simulink model "AUAV3_WITH_SLUGS_SENSOR_AND_CONTROLLER"  (Simulink 8.5)
settings: Solver=FixedStepDiscrete  StartTime=0.0  StopTime=10.0  FixedStep=T  RelTol=1e-3
PreLoadFcn:
  | T = 0.0025;
  | MavlinkBus;
  | 
  | % Baro Altitude Computation
  | % =========================
  | basePressure = 98192.64;
  | baseTemp = 288.215;
  | lapseRate = -0.00198122;
  | baseHeight = 0;
  | 
  | mcuInit
values from neighbouring files (symbols this model uses):
  apSampleTime = 0.01    [mcuInit.m]
  latlong_WP = 1    [mcuInit.m]
  mavlink_gps_raw_int_t = Simulink.Bus    [MavlinkBus.m]    (also in MavlinkBusMarcello.m)
  mavlink_raw_imu_t = Simulink.Bus    [MavlinkBus.m]    (also in MavlinkBusMarcello.m)
  mavlink_scaled_pressure_t = Simulink.Bus    [MavlinkBus.m]    (also in MavlinkBusMarcello.m)
  mavlink_sys_status_t = Simulink.Bus    [MavlinkBus.m]    (also in MavlinkBusMarcello.m)
  Xpoints = [0 0]    [mcuInit.m]
  Ypoints = [0 0]    [mcuInit.m]
  Zpoints = [0 0]    [mcuInit.m]
undefined symbols (not defined in the file or in its folder): A0, A14, A15, A2, A3, A5, A6, accBiasRateLimit, altLatLon, B0, bankCommandLimit, barAdjust, baroCutoff, baroCutTemp, C3, cubeAccelGain16405, cubeGyroGain16405, cubeMagGain16405, D0, D11, D13, D8, daLimit, data, daTrimMax, daTrimMin, deLimit, deTrimMax, deTrimMin, drLimit, drTrimMax, drTrimMin, dtLimit, dtTrimMax, dtTrimMin, F2, F3, G0, G15, gaind, GS_location, gyroBiasRateLimit, IC1max, IPStar, ISA_g, maxAcc, MaxDwnPthStar, maxDynPressure, maxEta, OC1max, P112, P127, P16, P21, P30, P31, P51, P64, P72, P75 ... (+39)
undefined symbols (not defined in the file): baroOffset, baroScale, barTGain1, barTGain2, barTMean1, barTMean2, bda, bde, bdr, bdt, bICda, bICde, bICdr, bICdt, derivativesConstant, lowRateSensorCutoff, mainSensorCutoff, mda, mde, mdr, mdt, mICda, mICde, mICdr, mICdt, pitotOffset, pitotScale, pitTGain1, pitTGain2, pitTMean1, pitTMean2, powerOffset, powerScale, pressureSensorCutoff, tempOffset, tempScale, vzCutoff, xCutoff, yCutoff
libraries: MCHP_Blockset x147, simulink x78, SLUGS_Library x31, aerolibconvert2 x6, aerolibutil x4, aerolibtransform2 x3, dspmtrx3 x2, aerolibobsolete x2
(part 12 of 12)

== matlab function Sensor Data [updated 4.28.16]/Sensor Suite/ADIS16405 Signal Cond /3D Tustin Lowpass, Auto Initial Condition/Embedded MATLAB Function1 ==
  data: u input double; y output double; T input double; f input double
function y = fcn(u,T,f)
% This block supports an embeddable subset of the MATLAB language.
% See the help menu for details. 

persistent a
persistent b
persistent y_km1
persistent u_km1
if isempty(a)
    %tf = [T*omega/(2+T*omega) T*omega/(2+T*omega)],[1 (T*omega-2)/(T*omega+2)]
    %tf = [a a],[1 -b]
    omega = 2*pi*f;
    a=T*omega/(2+T*omega);
    b=-(T*omega-2)/(T*omega+2);
    y_km1=u;
    u_km1=u;
end

y = a*(u+u_km1)+b*y_km1;
y_km1=y;
u_km1=u;

== matlab function Trim Vals [updated 4.28.16]/Control Surface Input/2 sec  tau/Embedded MATLAB Function ==
  data: u input double; y output double; T input double; f input double
function y = fcn(u,T,f)
% This block supports an embeddable subset of the MATLAB language.
% See the help menu for details. 

persistent a
persistent b
persistent y_km1
persistent u_km1
if isempty(a)
    %tf = [T*omega/(2+T*omega) T*omega/(2+T*omega)],[1 (T*omega-2)/(T*omega+2)]
    %tf = [a a],[1 -b]
    omega = 2*pi*f;
    a=T*omega/(2+T*omega);
    b=-(T*omega-2)/(T*omega+2);
    y_km1=u;
    u_km1=u;
end

y = a*(u+u_km1)+b*y_km1;
y_km1=y;
u_km1=u;

== matlab function Trim Vals [updated 4.28.16]/Control Surface Input/2 sec  tau1/Embedded MATLAB Function ==
  data: u input double; y output double; T input double; f input double
function y = fcn(u,T,f)
% This block supports an embeddable subset of the MATLAB language.
% See the help menu for details. 

persistent a
persistent b
persistent y_km1
persistent u_km1
if isempty(a)
    %tf = [T*omega/(2+T*omega) T*omega/(2+T*omega)],[1 (T*omega-2)/(T*omega+2)]
    %tf = [a a],[1 -b]
    omega = 2*pi*f;
    a=T*omega/(2+T*omega);
    b=-(T*omega-2)/(T*omega+2);
    y_km1=u;
    u_km1=u;
end

y = a*(u+u_km1)+b*y_km1;
y_km1=y;
u_km1=u;

== matlab function Sensor Data [updated 4.28.16]/Sensor Suite/ADIS16405 Signal Cond /3D Tustin Lowpass, Auto Initial Condition/Embedded MATLAB Function2 ==
  data: u input double; y output double; T input double; f input double
function y = fcn(u,T,f)
% This block supports an embeddable subset of the MATLAB language.
% See the help menu for details. 

persistent a
persistent b
persistent y_km1
persistent u_km1
if isempty(a)
    %tf = [T*omega/(2+T*omega) T*omega/(2+T*omega)],[1 (T*omega-2)/(T*omega+2)]
    %tf = [a a],[1 -b]
    omega = 2*pi*f;
    a=T*omega/(2+T*omega);
    b=-(T*omega-2)/(T*omega+2);
    y_km1=u;
    u_km1=u;
end

y = a*(u+u_km1)+b*y_km1;
y_km1=y;
u_km1=u;

== matlab function Trim Vals [updated 4.28.16]/Mean Filter the Transition/Buffer Failsafe Channel ==
  data: latest input double; history output double
function history = bufferICValues(latest)
% This block supports an embeddable subset of the MATLAB language.
% See the help menu for details. 

persistent oldValues;

if isempty(oldValues)
    oldValues = uint16([0 0 0 0 0 0 0]);
end

history = uint16([0 0 0 0 0 0 0]);

for i=7:-1:2
    oldValues(i) = oldValues(i-1);
	history(i) = oldValues(i-1);
end
	
oldValues(1) = latest;
history(1) = latest;

== matlab function Sensor Data [updated 4.28.16]/Sensor Suite/ADIS16405 Signal Cond /3D Tustin Lowpass, Auto Initial Condition/myMux Fun ==
  data: u1 input double; y output double; u2 input double; u3 input double
function y = myMux3(u1, u2, u3)
% This block supports an embeddable subset of the MATLAB language.
% See the help menu for details. 

y = [u1(1); u2(1); u3(1)];

== matlab function Sensor Data [updated 4.28.16]/Sensor Suite/ADIS16405 Signal Cond /3D Tustin Lowpass, Auto Initial Condition1/Embedded MATLAB Function ==
  data: u input double; y output double; T input double; f input double
function y = fcn(u,T,f)
% This block supports an embeddable subset of the MATLAB language.
% See the help menu for details. 

persistent a
persistent b
persistent y_km1
persistent u_km1
if isempty(a)
    %tf = [T*omega/(2+T*omega) T*omega/(2+T*omega)],[1 (T*omega-2)/(T*omega+2)]
    %tf = [a a],[1 -b]
    omega = 2*pi*f;
    a=T*omega/(2+T*omega);
    b=-(T*omega-2)/(T*omega+2);
    y_km1=u;
    u_km1=u;
end

y = a*(u+u_km1)+b*y_km1;
y_km1=y;
u_km1=u;

== matlab function Sensor Data [updated 4.28.16]/Sensor Suite/ADIS16405 Signal Cond /3D Tustin Lowpass, Auto Initial Condition1/Embedded MATLAB Function1 ==
  data: u input double; y output double; T input double; f input double
function y = fcn(u,T,f)
% This block supports an embeddable subset of the MATLAB language.
% See the help menu for details. 

persistent a
persistent b
persistent y_km1
persistent u_km1
if isempty(a)
    %tf = [T*omega/(2+T*omega) T*omega/(2+T*omega)],[1 (T*omega-2)/(T*omega+2)]
    %tf = [a a],[1 -b]
    omega = 2*pi*f;
    a=T*omega/(2+T*omega);
    b=-(T*omega-2)/(T*omega+2);
    y_km1=u;
    u_km1=u;
end

y = a*(u+u_km1)+b*y_km1;
y_km1=y;
u_km1=u;

== matlab function Sensor Data [updated 4.28.16]/Sensor Suite/ADIS16405 Signal Cond /3D Tustin Lowpass, Auto Initial Condition1/Embedded MATLAB Function2 ==
  data: u input double; y output double; T input double; f input double
function y = fcn(u,T,f)
% This block supports an embeddable subset of the MATLAB language.
% See the help menu for details. 

persistent a
persistent b
persistent y_km1
persistent u_km1
if isempty(a)
    %tf = [T*omega/(2+T*omega) T*omega/(2+T*omega)],[1 (T*omega-2)/(T*omega+2)]
    %tf = [a a],[1 -b]
    omega = 2*pi*f;
    a=T*omega/(2+T*omega);
    b=-(T*omega-2)/(T*omega+2);
    y_km1=u;
    u_km1=u;
end

y = a*(u+u_km1)+b*y_km1;
y_km1=y;
u_km1=u;

== matlab function Sensor Data [updated 4.28.16]/Sensor Suite/ADIS16405 Signal Cond /3D Tustin Lowpass, Auto Initial Condition1/myMux Fun ==
  data: u1 input double; y output double; u2 input double; u3 input double
function y = myMux3(u1, u2, u3)
% This block supports an embeddable subset of the MATLAB language.
% See the help menu for details. 

y = [u1(1); u2(1); u3(1)];

== matlab function Sensor Data [updated 4.28.16]/Sensor Suite/ADIS16405 Signal Cond /3D Tustin Lowpass, Auto Initial Condition2/Embedded MATLAB Function ==
  data: u input double; y output double; T input double; f input double
function y = fcn(u,T,f)
% This block supports an embeddable subset of the MATLAB language.
% See the help menu for details. 

persistent a
persistent b
persistent y_km1
persistent u_km1
if isempty(a)
    %tf = [T*omega/(2+T*omega) T*omega/(2+T*omega)],[1 (T*omega-2)/(T*omega+2)]
    %tf = [a a],[1 -b]
    omega = 2*pi*f;
    a=T*omega/(2+T*omega);
    b=-(T*omega-2)/(T*omega+2);
    y_km1=u;
    u_km1=u;
end

y = a*(u+u_km1)+b*y_km1;
y_km1=y;
u_km1=u;

== matlab function Sensor Data [updated 4.28.16]/Sensor Suite/ADIS16405 Signal Cond /3D Tustin Lowpass, Auto Initial Condition2/Embedded MATLAB Function1 ==
  data: u input double; y output double; T input double; f input double
function y = fcn(u,T,f)
% This block supports an embeddable subset of the MATLAB language.
% See the help menu for details. 

persistent a
persistent b
persistent y_km1
persistent u_km1
if isempty(a)
    %tf = [T*omega/(2+T*omega) T*omega/(2+T*omega)],[1 (T*omega-2)/(T*omega+2)]
    %tf = [a a],[1 -b]
    omega = 2*pi*f;
    a=T*omega/(2+T*omega);
    b=-(T*omega-2)/(T*omega+2);
    y_km1=u;
    u_km1=u;
end

y = a*(u+u_km1)+b*y_km1;
y_km1=y;
u_km1=u;

== matlab function Sensor Data [updated 4.28.16]/Sensor Suite/ADIS16405 Signal Cond /3D Tustin Lowpass, Auto Initial Condition2/Embedded MATLAB Function2 ==
  data: u input double; y output double; T input double; f input double
function y = fcn(u,T,f)
% This block supports an embeddable subset of the MATLAB language.
% See the help menu for details. 

persistent a
persistent b
persistent y_km1
persistent u_km1
if isempty(a)
    %tf = [T*omega/(2+T*omega) T*omega/(2+T*omega)],[1 (T*omega-2)/(T*omega+2)]
    %tf = [a a],[1 -b]
    omega = 2*pi*f;
    a=T*omega/(2+T*omega);
    b=-(T*omega-2)/(T*omega+2);
    y_km1=u;
    u_km1=u;
end

y = a*(u+u_km1)+b*y_km1;
y_km1=y;
u_km1=u;

== matlab function Sensor Data [updated 4.28.16]/Sensor Suite/ADIS16405 Signal Cond /3D Tustin Lowpass, Auto Initial Condition2/myMux Fun ==
  data: u1 input double; y output double; u2 input double; u3 input double
function y = myMux3(u1, u2, u3)
% This block supports an embeddable subset of the MATLAB language.
% See the help menu for details. 

y = [u1(1); u2(1); u3(1)];

== matlab function Sensor Data [updated 4.28.16]/Sensor Suite/If no HIL then Read all the Sensors/Embedded MATLAB Function ==
  data: u input double; y output double
function y = averageADC(u)
% This block supports an embeddable subset of the MATLAB language.
% See the help menu for details. 

y = (u(1)+ u(2) + u(3) + u(4) + u(5))*0.20;

== matlab function Sensor Data [updated 4.28.16]/Sensor Suite/If no HIL then Read all the Sensors/Embedded MATLAB Function1 ==
  data: u input double; y output double
function y = averageADC(u)
% This block supports an embeddable subset of the MATLAB language.
% See the help menu for details. 

y = (u(1)+ u(2) + u(3) + u(4) + u(5))*0.20;

== matlab function Sensor Data [updated 4.28.16]/Sensor Suite/If no HIL then Read all the Sensors/Embedded MATLAB Function2 ==
  data: u input double; y output double
function y = averageADC(u)
% This block supports an embeddable subset of the MATLAB language.
% See the help menu for details. 

y = (u(1)+ u(2) + u(3) + u(4) + u(5))*0.20;

== matlab function Sensor Data [updated 4.28.16]/Sensor Suite/If no HIL then Read all the Sensors/Embedded MATLAB Function3 ==
  data: u input double; y output double
function y = averageADC(u)
% This block supports an embeddable subset of the MATLAB language.
% See the help menu for details. 

y = (u(1)+ u(2) + u(3) + u(4) + u(5))*0.20;

== matlab function Sensor Data [updated 4.28.16]/Sensor Suite/If no HIL then Read all the Sensors/myMux Fun ==
  data: u1 input double; y output double; u2 input double; u3 input double; u4 input double
function y = myMux(u1, u2, u3, u4)
% This block supports an embeddable subset of the MATLAB language.
% See the help menu for details. 

y = [u1(1); u2(1); u3(1); u4(1)];

== matlab function Sensor Data [updated 4.28.16]/Sensor Suite/If no HIL then Read all the Sensors/myMux Fun4 ==
  data: u1 input double; y output double; u2 input double; u3 input double; u4 input double; u5 input double; u6 input double; u7 input double; u8 input double; u9 input double; u10 input double; u11 input double; u12 input double; u13 input double
function y = sensMux(u1, u2,u3,u4,u5,u6,u7,u8, u9, u10, u11, u12, u13)
% This block supports an embeddable subset of the MATLAB language.
% See the help menu for details. 

y = [u1(1); u2(1); u3(1); u4(1); u5(1); u6(1); u7(1); u8(1); u9(1); u10(1); u11(1); u12(1); u13(1)];

== matlab function Sensor Data [updated 4.28.16]/Sensor Suite/Low Pass Filtering,Temperature Compensation and Calibration/Baro Altimeter/Enables/Disables the Computation of initial Baro Bias ==
  data: tOut output double
function tOut = getTIni

persistent aveCount;
persistent tIni;

if isempty(aveCount)
    aveCount =1;
    tIni = 1;
end;

if aveCount < 2500
    aveCount = aveCount + 1;
end

if aveCount == 2500
    tIni =0;
    aveCount = aveCount + 1;
end

tOut = tIni;

%if aveCount > 500
%    tIni = 0;
%end

% if isempty(aveCount)
%     aveCount =1;
%     initBias = [0.0 0.0 0.0]';
% end;
%     
% if (aveCount<10)
%     initBias = initBias+ Raw;
%     bias = initBias/aveCount;
%     aveCount = aveCount +1;
% end;
% 
% if (aveCount == 10)
%     initBias = initBias/(aveCount-1);
%     aveCount = 100;
% end;
% 
% if (aveCount == 100)
%     bias = initBias;
% end;

== matlab function Sensor Data [updated 4.28.16]/Sensor Suite/Low Pass Filtering,Temperature Compensation and Calibration/Tustin Lowpass, Auto Initial Condition1/Embedded MATLAB Function ==
  data: u input double; y output double; T input double; f input double
function y = fcn(u,T,f)
% This block supports an embeddable subset of the MATLAB language.
% See the help menu for details. 

persistent a
persistent b
persistent y_km1
persistent u_km1
if isempty(a)
    %tf = [T*omega/(2+T*omega) T*omega/(2+T*omega)],[1 (T*omega-2)/(T*omega+2)]
    %tf = [a a],[1 -b]
    omega = 2*pi*f;
    a=T*omega/(2+T*omega);
    b=-(T*omega-2)/(T*omega+2);
    y_km1=u;
    u_km1=u;
end

y = a*(u+u_km1)+b*y_km1;
y_km1=y;
u_km1=u;

== matlab function Sensor Data [updated 4.28.16]/Sensor Suite/Low Pass Filtering,Temperature Compensation and Calibration/Tustin Lowpass, Auto Initial Condition2/Embedded MATLAB Function ==
  data: u input double; y output double; T input double; f input double
function y = fcn(u,T,f)
% This block supports an embeddable subset of the MATLAB language.
% See the help menu for details. 

persistent a
persistent b
persistent y_km1
persistent u_km1
if isempty(a)
    %tf = [T*omega/(2+T*omega) T*omega/(2+T*omega)],[1 (T*omega-2)/(T*omega+2)]
    %tf = [a a],[1 -b]
    omega = 2*pi*f;
    a=T*omega/(2+T*omega);
    b=-(T*omega-2)/(T*omega+2);
    y_km1=u;
    u_km1=u;
end

y = a*(u+u_km1)+b*y_km1;
y_km1=y;
u_km1=u;

== matlab function Sensor Data [updated 4.28.16]/Sensor Suite/Low Pass Filtering,Temperature Compensation and Calibration/Tustin Lowpass, Auto Initial Condition3/Embedded MATLAB Function ==
  data: u input double; y output double; T input double; f input double
function y = fcn(u,T,f)
% This block supports an embeddable subset of the MATLAB language.
% See the help menu for details. 

persistent a
persistent b
persistent y_km1
persistent u_km1
if isempty(a)
    %tf = [T*omega/(2+T*omega) T*omega/(2+T*omega)],[1 (T*omega-2)/(T*omega+2)]
    %tf = [a a],[1 -b]
    omega = 2*pi*f;
    a=T*omega/(2+T*omega);
    b=-(T*omega-2)/(T*omega+2);
    y_km1=u;
    u_km1=u;
end

y = a*(u+u_km1)+b*y_km1;
y_km1=y;
u_km1=u;

== matlab function Sensor Data [updated 4.28.16]/Sensor Suite/Low Pass Filtering,Temperature Compensation and Calibration/Tustin Lowpass, Auto Initial Condition4/Embedded MATLAB Function ==
  data: u input double; y output double; T input double; f input double
function y = fcn(u,T,f)
% This block supports an embeddable subset of the MATLAB language.
% See the help menu for details. 

persistent a
persistent b
persistent y_km1
persistent u_km1
if isempty(a)
    %tf = [T*omega/(2+T*omega) T*omega/(2+T*omega)],[1 (T*omega-2)/(T*omega+2)]
    %tf = [a a],[1 -b]
    omega = 2*pi*f;
    a=T*omega/(2+T*omega);
    b=-(T*omega-2)/(T*omega+2);
    y_km1=u;
    u_km1=u;
end

y = a*(u+u_km1)+b*y_km1;
y_km1=y;
u_km1=u;

== matlab function Sensor Data [updated 4.28.16]/Sensor Suite/myMux Fun ==
  data: u1 input double; y output double; u2 input double; u3 input double
function y = myMux3(u1, u2, u3)
% This block supports an embeddable subset of the MATLAB language.
% See the help menu for details. 

y = [u1(1); u2(1); u3(1)];

== matlab function Sensor Data [updated 4.28.16]/Sensor Suite/myMux Fun1 ==
  data: u1 input double; y output double; u2 input double; u3 input double; u4 input double
function y = myMux31(u1, u2, u3, u4)
% This block supports an embeddable subset of the MATLAB language.
% See the help menu for details. 

y = [u1(1); u2(1); u3(1); u4(1)];

== matlab function Inner Loop/ Navigation/Navigation Encaps [updated 4.28.16]/Navigation/Normal WP Navigation/Get Frenet/Compute Frenet/Select N Terms ==
  data: T input double; N output double
function N = getN(T)
% This block supports an embeddable subset of the MATLAB language.
% See the help menu for details. 

N = [-T(2); T(1); 0];

== matlab function Inner Loop/ Navigation/Navigation Encaps [updated 4.28.16]/Navigation/Normal WP Navigation/Get Frenet/Compute Frenet/Normalize Vector /Vector Norm/dsPIC_SQRT/negprotect ==
  data: val input double; zpVal output double
function zpVal = negProt(val)
% This block supports an embeddable subset of the MATLAB language.
% See the help menu for details. 

if val >= single(0.001)
    zpVal = val;
else
    zpVal = single(0.001);
end

== matlab function Inner Loop/ Navigation/Navigation Encaps [updated 4.28.16]/Navigation/Normal WP Navigation/Get Frenet/get WP Coord from Index1/Get WP from idx SIM/Zero out Z1 ==
  data: y output double; idx input double; vect input double
function y = GetVectorElement(idx , vect)
% This block supports an embeddable subset of the MATLAB language.
% See the help menu for details. 

y = vect(idx);

== matlab function Inner Loop/ Navigation/Navigation Encaps [updated 4.28.16]/Navigation/Normal WP Navigation/Get Frenet/get WP Coord from Index1/Get WP from idx SIM/Zero out Z2 ==
  data: y output double; idx input double; vect input double
function y = GetVectorElement(idx , vect)
% This block supports an embeddable subset of the MATLAB language.
% See the help menu for details. 

y = vect(idx);

== matlab function Inner Loop/ Navigation/Navigation Encaps [updated 4.28.16]/Navigation/Normal WP Navigation/Get Frenet/get WP Coord from Index1/Get WP from idx SIM/Zero out Z3 ==
  data: y output double; idx input double; vect input double
function y = GetVectorElement(idx , vect)
% This block supports an embeddable subset of the MATLAB language.
% See the help menu for details. 

y = vect(idx);

== matlab function Inner Loop/ Navigation/Navigation Encaps [updated 4.28.16]/Navigation/Normal WP Navigation/Get Frenet/get WP Coord from Index2/Get WP from idx SIM/Zero out Z1 ==
  data: y output double; idx input double; vect input double
function y = GetVectorElement(idx , vect)
% This block supports an embeddable subset of the MATLAB language.
% See the help menu for details. 

y = vect(idx);

== matlab function Inner Loop/ Navigation/Navigation Encaps [updated 4.28.16]/Navigation/Normal WP Navigation/Get Frenet/get WP Coord from Index2/Get WP from idx SIM/Zero out Z2 ==
  data: y output double; idx input double; vect input double
function y = GetVectorElement(idx , vect)
% This block supports an embeddable subset of the MATLAB language.
% See the help menu for details. 

y = vect(idx);

== matlab function Inner Loop/ Navigation/Navigation Encaps [updated 4.28.16]/Navigation/Normal WP Navigation/Get Frenet/get WP Coord from Index2/Get WP from idx SIM/Zero out Z3 ==
  data: y output double; idx input double; vect input double
function y = GetVectorElement(idx , vect)
% This block supports an embeddable subset of the MATLAB language.
% See the help menu for details. 

y = vect(idx);

== matlab function Inner Loop/ Navigation/Navigation Encaps [updated 4.28.16]/Navigation/Normal WP Navigation/On WP Enable/Subsystem/Compute Frenet/Normalize Vector/Vector Norm/dsPIC_SQRT/negprotect ==
  data: val input double; zpVal output double
function zpVal = negProt(val)
% This block supports an embeddable subset of the MATLAB language.
% See the help menu for details. 

if val >= single(0.001)
    zpVal = val;
else
    zpVal = single(0.001);
end

== matlab function Inner Loop/ Navigation/Navigation Encaps [updated 4.28.16]/Navigation/Normal WP Navigation/On WP Enable/Subsystem/Compute Frenet/Select N Terms ==
  data: T input double; N output double
function N = getN(T)
% This block supports an embeddable subset of the MATLAB language.
% See the help menu for details. 

N = [-T(2); T(1); 0];

== matlab function Inner Loop/ Navigation/Navigation Encaps [updated 4.28.16]/Navigation/Normal WP Navigation/On WP Enable/Subsystem/Compute Frenet/Normalize Vector /Vector Norm/dsPIC_SQRT/negprotect ==
  data: val input double; zpVal output double
function zpVal = negProt(val)
% This block supports an embeddable subset of the MATLAB language.
% See the help menu for details. 

if val >= single(0.001)
    zpVal = val;
else
    zpVal = single(0.001);
end

== matlab function Inner Loop/ Navigation/Navigation Encaps [updated 4.28.16]/Navigation/Normal WP Navigation/On WP Enable/Subsystem/get WP Coord from Index/Get WP from idx SIM/Zero out Z1 ==
  data: y output double; idx input double; vect input double
function y = GetVectorElement(idx , vect)
% This block supports an embeddable subset of the MATLAB language.
% See the help menu for details. 

y = vect(idx);

== matlab function Inner Loop/ Navigation/Navigation Encaps [updated 4.28.16]/Navigation/Normal WP Navigation/On WP Enable/Subsystem/get WP Coord from Index/Get WP from idx SIM/Zero out Z2 ==
  data: y output double; idx input double; vect input double
function y = GetVectorElement(idx , vect)
% This block supports an embeddable subset of the MATLAB language.
% See the help menu for details. 

y = vect(idx);

== matlab function Inner Loop/ Navigation/Navigation Encaps [updated 4.28.16]/Navigation/Normal WP Navigation/On WP Enable/Subsystem/get WP Coord from Index/Get WP from idx SIM/Zero out Z3 ==
  data: y output double; idx input double; vect input double
function y = GetVectorElement(idx , vect)
% This block supports an embeddable subset of the MATLAB language.
% See the help menu for details. 

y = vect(idx);

== matlab function Inner Loop/ Navigation/Navigation Encaps [updated 4.28.16]/Navigation/Normal WP Navigation/On WP Enable/Subsystem/get WP Coord from Index1/Get WP from idx SIM/Zero out Z1 ==
  data: y output double; idx input double; vect input double
function y = GetVectorElement(idx , vect)
% This block supports an embeddable subset of the MATLAB language.
% See the help menu for details. 

y = vect(idx);

== matlab function Inner Loop/ Navigation/Navigation Encaps [updated 4.28.16]/Navigation/Normal WP Navigation/On WP Enable/Subsystem/get WP Coord from Index1/Get WP from idx SIM/Zero out Z2 ==
  data: y output double; idx input double; vect input double
function y = GetVectorElement(idx , vect)
% This block supports an embeddable subset of the MATLAB language.
% See the help menu for details. 

y = vect(idx);

== matlab function Inner Loop/ Navigation/Navigation Encaps [updated 4.28.16]/Navigation/Normal WP Navigation/On WP Enable/Subsystem/get WP Coord from Index1/Get WP from idx SIM/Zero out Z3 ==
  data: y output double; idx input double; vect input double
function y = GetVectorElement(idx , vect)
% This block supports an embeddable subset of the MATLAB language.
% See the help menu for details. 

y = vect(idx);

== matlab function Inner Loop/ Navigation/Navigation Encaps [updated 4.28.16]/Navigation/Normal WP Navigation/Vector Norm/dsPIC_SQRT/negprotect ==
  data: val input double; zpVal output double
function zpVal = negProt(val)
% This block supports an embeddable subset of the MATLAB language.
% See the help menu for details. 

if val >= single(0.001)
    zpVal = val;
else
    zpVal = single(0.001);
end

== matlab function Inner Loop/ Navigation/Navigation Encaps [updated 4.28.16]/Navigation/RTB/Follow Mobile Navigation/Vector Norm/dsPIC_SQRT/negprotect ==
  data: val input double; zpVal output double
function zpVal = negProt(val)
% This block supports an embeddable subset of the MATLAB language.
% See the help menu for details. 

if val >= single(0.001)
    zpVal = val;
else
    zpVal = single(0.001);
end
